simulink library "INT_InjCrv_MI1"  (R2016b)
settings: Solver=VariableStepAuto  StartTime=0.0  StopTime=10.0  RelTol=1e-3
settings Model: Creator=mayongchao  LastModifiedBy=mayongchao

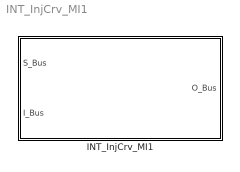
== system INT_InjCrv_MI1 ==
  INT_InjCrv_MI1 : Subsystem

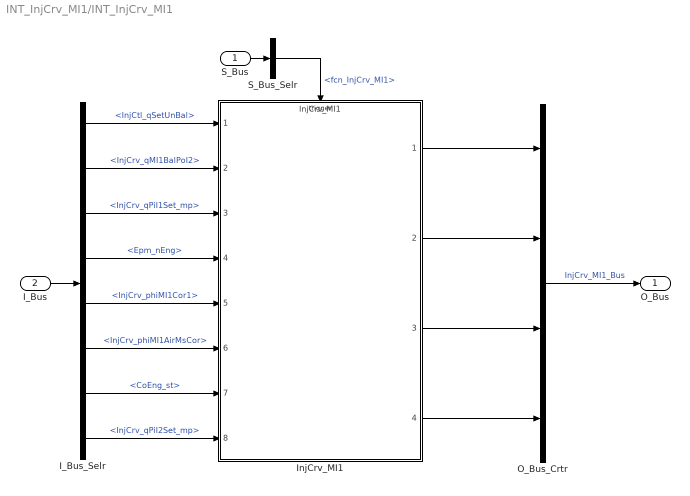
== system INT_InjCrv_MI1/INT_InjCrv_MI1 ==
  S_Bus : Inport
  I_Bus : Inport  Port=2
  I_Bus_Selr : BusSelector  OutputSignals=InjCtl_qSetUnBal,InjCrv_qMI1BalPoI2,InjCrv_qPiI1Set_mp,Epm_nEng,InjCrv_phiMI1Cor1,InjCrv_phiMI1AirMsCor,CoEng_st,InjCrv_qPiI2Set_mp
  InjCrv_MI1 : ModelReference  ModelNameDialog=InjCrv_MI1  SimulationMode=Normal  ModelReferenceVersion=1.46  TriggerPortName=function  TriggerPortTriggerType=function-call  TriggerPortStatesWhenEnabling=held
  O_Bus_Crtr : BusCreator  Inputs=4
  S_Bus_Selr : BusSelector  OutputSignals=fcn_InjCrv_MI1
  O_Bus : Outport
  wires:
  S_Bus_Selr/1 -> InjCrv_MI1/Trigger  "<fcn_InjCrv_MI1>"
  S_Bus/1 -> S_Bus_Selr/1
  I_Bus/1 -> I_Bus_Selr/1
  I_Bus_Selr/1 -> InjCrv_MI1/1  "<InjCtl_qSetUnBal>"
  I_Bus_Selr/2 -> InjCrv_MI1/2  "<InjCrv_qMI1BalPoI2>"
  I_Bus_Selr/3 -> InjCrv_MI1/3  "<InjCrv_qPiI1Set_mp>"
  I_Bus_Selr/4 -> InjCrv_MI1/4  "<Epm_nEng>"
  I_Bus_Selr/5 -> InjCrv_MI1/5  "<InjCrv_phiMI1Cor1>"
  I_Bus_Selr/6 -> InjCrv_MI1/6  "<InjCrv_phiMI1AirMsCor>"
  I_Bus_Selr/7 -> InjCrv_MI1/7  "<CoEng_st>"
  I_Bus_Selr/8 -> InjCrv_MI1/8  "<InjCrv_qPiI2Set_mp>"
  O_Bus_Crtr/1 -> O_Bus/1  "InjCrv_MI1_Bus"
  InjCrv_MI1/1 -> O_Bus_Crtr/1
  InjCrv_MI1/2 -> O_Bus_Crtr/2
  InjCrv_MI1/3 -> O_Bus_Crtr/3
  InjCrv_MI1/4 -> O_Bus_Crtr/4
